simulink model "OpenLoop_Test"  (R2023b)
settings: Solver=VariableStepAuto  StartTime=0.0  StopTime=10.0  RelTol=1e-6
libraries: cstblocks x6
settings Model: Creator=bolee  LastModifiedBy=bolee

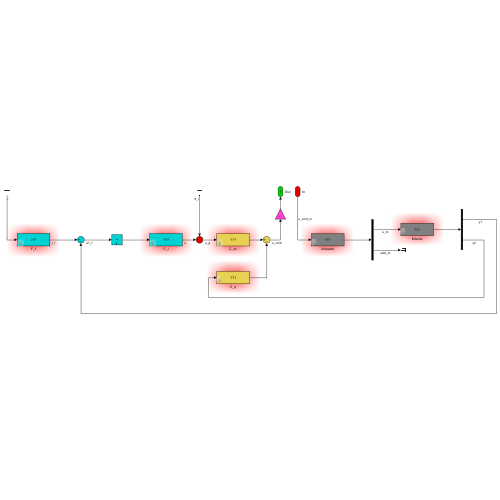
[thumbnail: Simulink's stored preview of the top-level diagram]
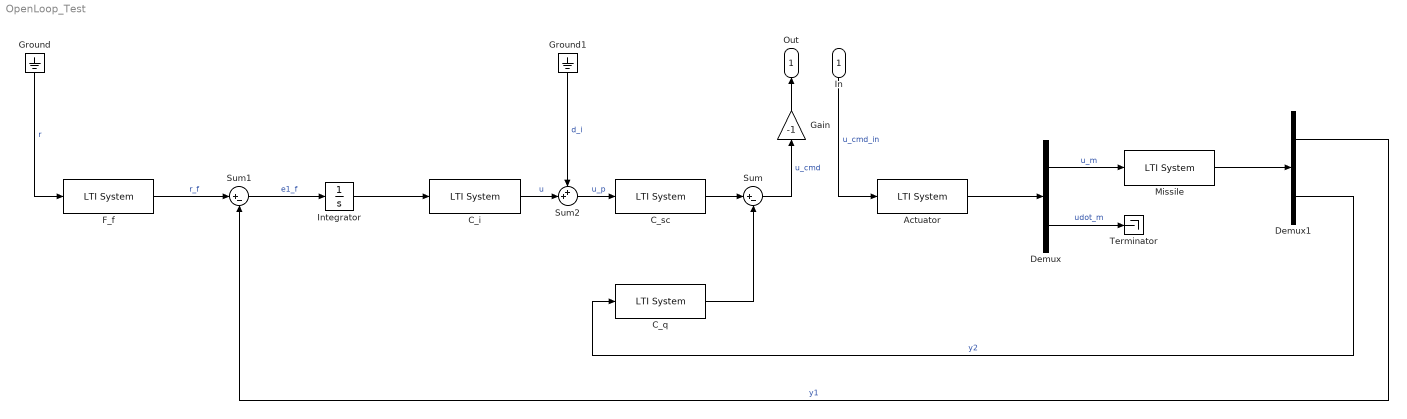
== system OpenLoop_Test ==
  In : Inport
  Actuator : cstblocks/LTI System  sys=G_a  IC=[]  PadeOrder=0
  C_i : cstblocks/LTI System  sys=C_i  IC=[]  PadeOrder=0
  C_q : cstblocks/LTI System  sys=C_q  IC=[]  PadeOrder=0
  C_sc : cstblocks/LTI System  sys=C_sc  IC=[]  PadeOrder=0
  Demux : Demux  Outputs=2
  Demux1 : Demux  Outputs=2
  F_f : cstblocks/LTI System  sys=F_f  IC=[]  PadeOrder=0
  Gain : Gain  Gain=-1
  Ground : Ground
  Ground1 : Ground
  Integrator : Integrator
  Missile : cstblocks/LTI System  sys=G_m  IC=[]  PadeOrder=0
  Sum : Sum  Inputs=|+-
  Sum1 : Sum  Inputs=|+-
  Sum2 : Sum  Inputs=++|
  Terminator : Terminator
  Out : Outport
  wires:
  Actuator/1 -> Demux/1
  Demux/1 -> Missile/1  "u_m"
  Demux/2 -> Terminator/1  "udot_m"
  Missile/1 -> Demux1/1
  Demux1/1 -> Sum1/2  "y1"
  C_q/1 -> Sum/2
  Demux1/2 -> C_q/1  "y2"
  C_sc/1 -> Sum/1
  Integrator/1 -> C_i/1
  Ground/1 -> F_f/1  "r"
  F_f/1 -> Sum1/1  "r_f"
  Sum1/1 -> Integrator/1  "e1_f"
  Sum2/1 -> C_sc/1  "u_p"
  C_i/1 -> Sum2/2  "u"
  Ground1/1 -> Sum2/1  "d_i"
  Sum/1 -> Gain/1  "u_cmd"
  Gain/1 -> Out/1
  In/1 -> Actuator/1  "u_cmd_in"
